simulink model "CruiseControlModel"  (R2024b)
settings: Solver=VariableStepAuto  StartTime=0.0  StopTime=10.0  RelTol=1e-3
settings Model: Creator=HP  LastModifiedBy=HP

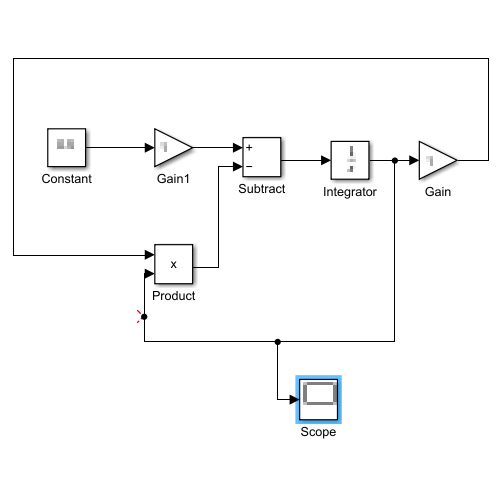
[thumbnail: Simulink's stored preview of the top-level diagram]
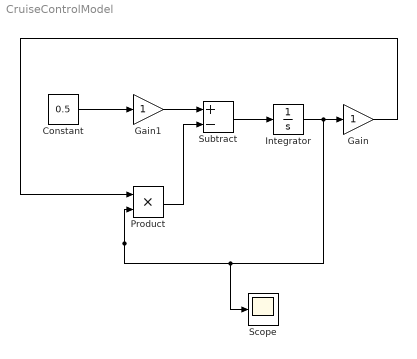
== system CruiseControlModel ==
  Constant : Constant  Value=0.5
  Gain : Gain
  Gain1 : Gain
  Integrator : Integrator
  Product : Product
  Scope : Scope
  Subtract : Sum  Inputs=+-
  wires:
  Constant/1 -> Gain1/1
  Subtract/1 -> Integrator/1
  Gain1/1 -> Subtract/1
  Product/1 -> Subtract/2
  Gain/1 -> Product/1
  Integrator/1 -> Gain/1, Scope/1, Product/2
